simulink model "CS_SKILL_7_AM_SPECTRUM"  (R2023b)
settings: Solver=VariableStepAuto  StartTime=0.0  StopTime=5  RelTol=1e-3
libraries: commanapbnd3 x1, dspxfrm3 x1, dspsrcs4 x1
settings Model: Creator=dev22  LastModifiedBy=dev22

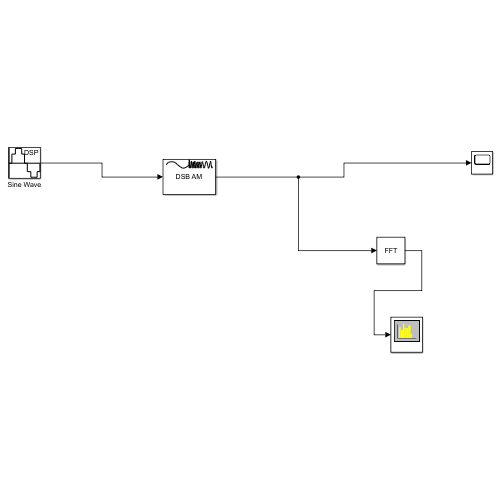
[thumbnail: Simulink's stored preview of the top-level diagram]
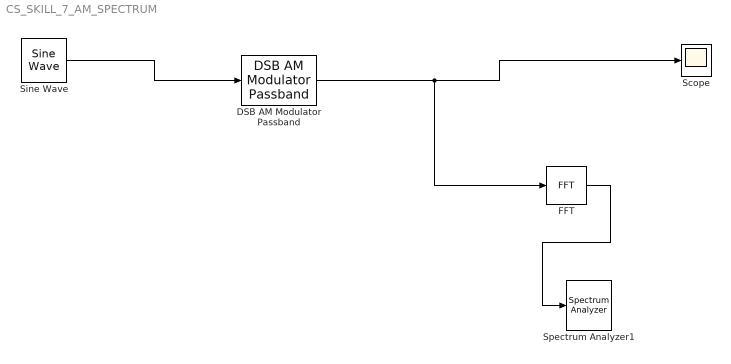
== system CS_SKILL_7_AM_SPECTRUM ==
  DSB AM Modulator Passband : commanapbnd3/DSB AM Modulator Passband  Fc=200  Ph=0  Offset=1
  FFT : dspxfrm3/FFT  FFTImplementation=Auto  CompMethod=Table lookup  TableOpt=NEW  TableOptActive=Speed  BitRevOrder=off  Normalize=off  InheritFFTLength=on  FFTLength=64  WrapInput=on  roundingMode=Floor  overflowMode=off  firstCoeffDataTypeStr=Inherit: Same word length as input  firstCoeffLastDataTypeStr=Inherit: Same word length as input  outputMin=[]  outputMax=[]
  Scope : Scope
  Sine Wave : dspsrcs4/Sine Wave  Amplitude=1  Frequency=10  Phase=0  SampleMode=Discrete  OutComplex=Real  CompMethod=Trigonometric fcn  TableSize=Speed  SampleTime=1/1000  SamplesPerFrame=1  ResetState=Restart at time zero  OutputFrames=off  dataType=double  wordLen=16  udDataType=sfix(16)  fracBitsMode=Best precision  numFracBits=15  OutDataTypeStr=double  LastOutDataTypeStr=double
  Spectrum Analyzer1 : SpectrumAnalyzer  WindowPosition=[1.000000,49.000000,1536.000000,793.000000,]  ScopeFrameLocation=window  YLimits=[-142.43276511,-16.10435046]
  wires:
  Sine Wave/1 -> DSB AM Modulator Passband/1
  DSB AM Modulator Passband/1 -> FFT/1, Scope/1
  FFT/1 -> Spectrum Analyzer1/1
